simulink model "fuzzycontroller"  (R2016b)
settings: Solver=FixedStepAuto  StartTime=0.0  StopTime=100  FixedStep=.01  RelTol=1e-3
libraries: fuzblock x2, simulink x1
settings Model: Creator=user  LastModifiedBy=user

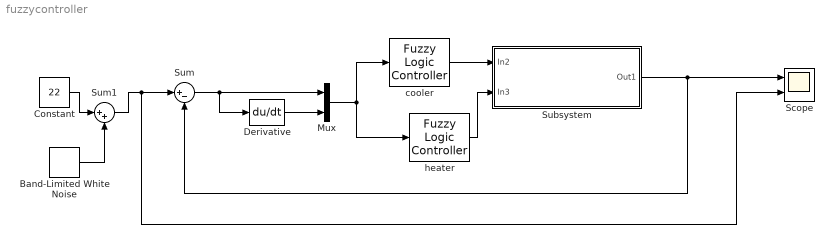
== system fuzzycontroller ==
  Band-Limited White Noise : simulink/Sources/Band-Limited White Noise  Cov=[0.1]  Ts=0.1  seed=[23341]
  Constant : Constant  Value=22
  Derivative : Derivative
  Mux : Mux  Inputs=2
  Scope : Scope  NumInputPorts=2
  Subsystem : Subsystem
  Sum : Sum  Inputs=|+-
  Sum1 : Sum  Inputs=|++
  cooler : fuzblock/Fuzzy Logic  Controller  fis='cooler1.fis'
  heater : fuzblock/Fuzzy Logic  Controller  fis='heater1.fis'
  wires:
  Subsystem/1(Out1) -> Sum/2, Scope/1
  Sum/1 -> Derivative/1, Mux/1
  cooler/1 -> Subsystem/1(In2)
  heater/1 -> Subsystem/2(In3)
  Sum1/1 -> Scope/2, Sum/1
  Derivative/1 -> Mux/2
  Mux/1 -> heater/1, cooler/1
  Constant/1 -> Sum1/1
  Band-Limited White Noise/1 -> Sum1/2

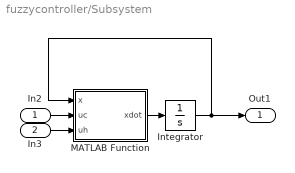
== system fuzzycontroller/Subsystem ==
  In2 : Inport
  In3 : Inport  Port=2
  Integrator : Integrator
  MATLAB Function : MATLAB Function  TreatAsAtomicUnit=on
  Out1 : Outport
  wires:
  MATLAB Function/1(xdot) -> Integrator/1
  Integrator/1 -> Out1/1, MATLAB Function/1(x)
  In3/1 -> MATLAB Function/3(uh)
  In2/1 -> MATLAB Function/2(uc)

== matlab function fuzzycontroller/Subsystem/MATLAB Function ==
  data: x input; xdot output; uc input; uh input
function xdot = fcn(x , uc ,uh)

xdot = -.1 *(x - 17) - .5 *uc + .5 * uh;
